simulink model "bane_masu_danpa"  (R2019a)
settings: Solver=VariableStepAuto  StartTime=0.0  StopTime=10.0  RelTol=1e-3
undefined symbols (not defined in the file): c, k, m
settings Model: Creator=robot  LastModifiedBy=robot

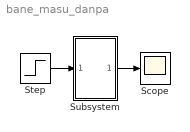
== system bane_masu_danpa ==
  Scope : Scope
  Step : Step  SampleTime=0
  Subsystem : Subsystem
  wires:
  Step/1 -> Subsystem/1(In1)
  Subsystem/1(Out1) -> Scope/1

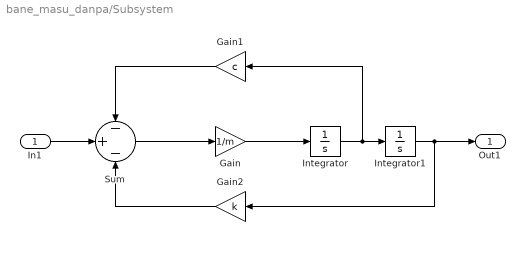
== system bane_masu_danpa/Subsystem ==
  In1 : Inport
  Gain : Gain  Gain=1/m
  Gain1 : Gain  Gain=c
  Gain2 : Gain  Gain=k
  Integrator : Integrator
  Integrator1 : Integrator
  Sum : Sum  Inputs=-+-
  Out1 : Outport
  wires:
  Gain/1 -> Integrator/1
  Integrator/1 -> Gain1/1, Integrator1/1
  Integrator1/1 -> Out1/1, Gain2/1
  Gain1/1 -> Sum/1
  In1/1 -> Sum/2
  Sum/1 -> Gain/1
  Gain2/1 -> Sum/3
